simulink model "harness_sensors_test"  (R2025a)
settings: Solver=VariableStepAuto  StartTime=0.0  StopTime=10.0  RelTol=1e-3
libraries: simulink x2
settings Model: Creator=Jackt  LastModifiedBy=Jackt

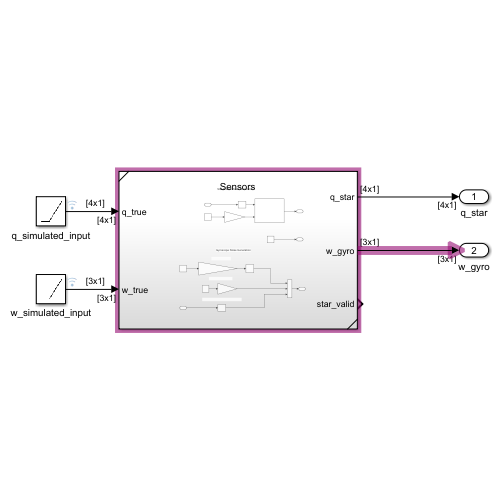
[thumbnail: Simulink's stored preview of the top-level diagram]
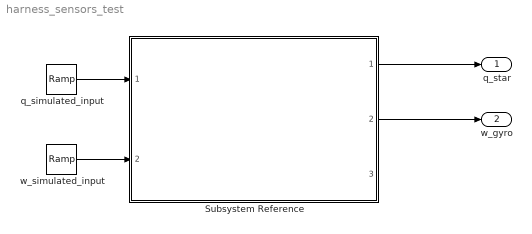
== system harness_sensors_test ==
  Subsystem Reference : Subsystem  ReferencedSubsystem=Sensors
  q_simulated_input : simulink/Sources/Ramp  slope=[-0.1; 0; 0.1; 0]  start=[0; 0; 0; 0]  InitialOutput=[1; 0; 0; 0]  VectorParams1D=off
  w_simulated_input : simulink/Sources/Ramp  slope=[1; 1; 0.5]  start=[0; 0.5; 0]  InitialOutput=[0; 0; 0]  VectorParams1D=off
  q_star : Outport
  w_gyro : Outport  Port=2
  wires:
  Subsystem Reference/1 -> q_star/1
  Subsystem Reference/2 -> w_gyro/1
  w_simulated_input/1 -> Subsystem Reference/2
  q_simulated_input/1 -> Subsystem Reference/1
